simulink model "Subsystem0"  (R2020b)
settings: Solver=VariableStepAuto  StartTime=0.0  StopTime=10.0  RelTol=1e-3
settings Model: Creator=Dell  LastModifiedBy=Dell
settings DataIOCC: SaveOutput=off  SaveTime=off

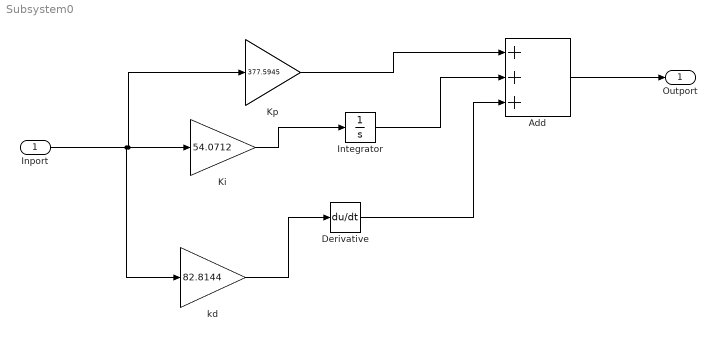
== system Subsystem0 ==
  Inport : Inport  OutDataTypeStr=double  PortDimensions=1  SampleTime=0
  Add : Sum  Inputs=+++
  Derivative : Derivative
  Integrator : Integrator
  Ki : Gain  Gain=54.0712
  Kp : Gain  Gain=377.5945
  kd : Gain  Gain=82.8144
  Outport : Outport  OutDataTypeStr=double  PortDimensions=1  SampleTime=0
  wires:
  Derivative/1 -> Add/3
  Inport/1 -> kd/1, Ki/1, Kp/1
  Add/1 -> Outport/1
  Kp/1 -> Add/1
  Integrator/1 -> Add/2
  Ki/1 -> Integrator/1
  kd/1 -> Derivative/1
